simulink model "project_task3"  (R2020b)
settings: Solver=ode4  StartTime=0.0  StopTime=1200  FixedStep=0.001  RelTol=1e-3
model workspace (MAT data in the model file):
  A = Simulink.Parameter
  A.Value = Simulink.data.Expression
  A.Value.ExpressionString = "(Iw*4.68)/(5*Kt*r)"
  A.DataType = 'auto'
  A.Dimensions = -1
  B = Simulink.Parameter
  B.Value = Simulink.data.Expression
  B.Value.ExpressionString = "(mt*r*4.68)/(5*Kt)"
  B.DataType = 'auto'
  B.Dimensions = -1
  C_prime = Simulink.Parameter
  C_prime.Value = Simulink.data.Expression
  C_prime.Value.ExpressionString = "(mt*10*r*4.68)/(5*Kt)"
  C_prime.DataType = 'auto'
  C_prime.Dimensions = -1
  D = Simulink.Parameter
  D.Value = Simulink.data.Expression
  D.Value.ExpressionString = "5*Kv/r"
  D.DataType = 'auto'
  D.Dimensions = -1
  Iw = Simulink.Parameter
  Iw.Value = Simulink.data.Expression
  Iw.Value.ExpressionString = "mw*r^2"
  Iw.DataType = 'auto'
  Iw.Dimensions = -1
  Kt = 0.0758
  Kv = 0.076
  mb = 0.4
  mc = 0.2
  mm = 0.34
  mt = Simulink.Parameter
  mt.Value = Simulink.data.Expression
  mt.Value.ExpressionString = "mc+mb+mw+mm"
  mt.DataType = 'auto'
  mt.Dimensions = -1
  mw = Simulink.Parameter
  mw.Value = Simulink.data.Expression
  mw.Value.ExpressionString = "0.5*r"
  mw.DataType = 'auto'
  mw.Dimensions = -1
  r = 0.39
  y_dot_desired = 0.5
libraries: eePwmGenerator x1, simulink_extras x1
settings Model: OrderedModelArguments=off  Creator=melih.turkseven  LastModifiedBy=berkt
settings SFSimCC: CustomCodeUndefinedFunction=UseInterfaceOnly

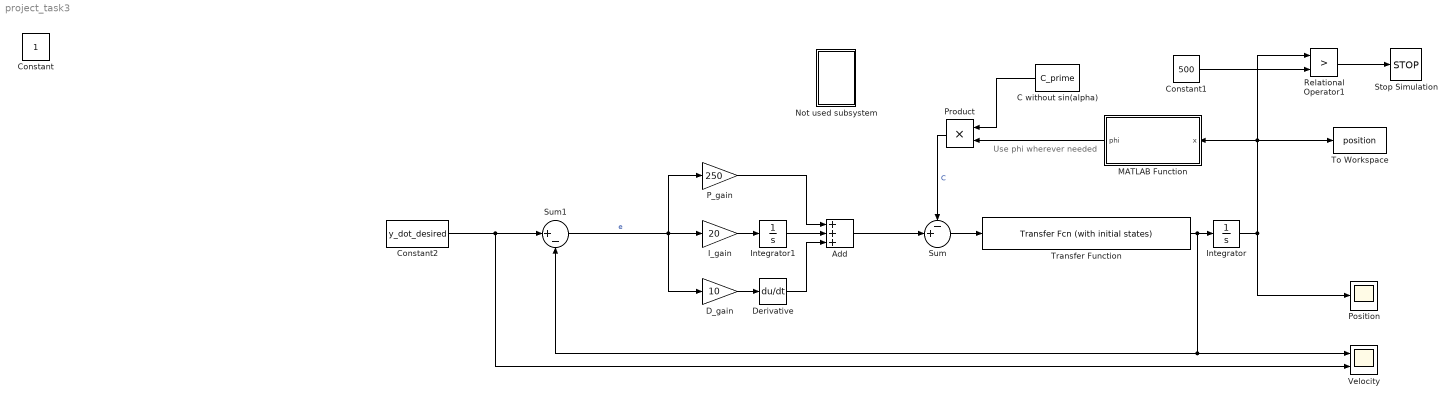
== system project_task3 ==
  note: Use phi wherever needed
  Add : Sum  Inputs=+++
  C without sin(alpha) : Constant  Value=C_prime
  Constant1 : Constant  Value=500
  Constant2 : Constant  Value=y_dot_desired
  D_gain : Gain  Gain=10
  Derivative : Derivative
  I_gain : Gain  Gain=20
  Integrator : Integrator
  Integrator1 : Integrator
  MATLAB Function : MATLAB Function  TreatAsAtomicUnit=on
  Not used subsystem : Subsystem
  P_gain : Gain  Gain=250
  Position : Scope
  Product : Product
  Relational Operator1 : RelationalOperator  Operator=>  OutDataTypeStr=boolean  RndMeth=Simplest
  Stop Simulation : Stop
  Sum : Sum  Inputs=-+|
  Sum1 : Sum  Inputs=|+-
  To Workspace : ToWorkspace  VariableName=position  SampleTime=-1
  Transfer Function : simulink_extras/Additional Linear/Transfer Fcn (with initial states)  N=[1]  D=[(A+B) D]  X0=0
  Velocity : Scope  NumInputPorts=2
  Constant : Constant  IOType=siggen
  wires:
  Transfer Function/1 -> Sum1/2, Velocity/1, Integrator/1
  MATLAB Function/1(phi) -> Product/2
  Relational Operator1/1 -> Stop Simulation/1
  Constant1/1 -> Relational Operator1/2
  Sum/1 -> Transfer Function/1
  C without sin(alpha)/1 -> Product/1
  Product/1 -> Sum/1  "C"
  Integrator/1 -> MATLAB Function/1(x), Relational Operator1/1, To Workspace/1, Position/1
  Constant2/1 -> Velocity/2, Sum1/1
  Sum1/1 -> P_gain/1, D_gain/1, I_gain/1  "e"
  I_gain/1 -> Integrator1/1
  D_gain/1 -> Derivative/1
  P_gain/1 -> Add/1
  Integrator1/1 -> Add/2
  Derivative/1 -> Add/3
  Add/1 -> Sum/2

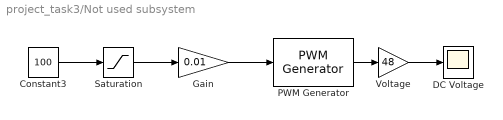
== system project_task3/Not used subsystem ==
  Constant3 : Constant  Value=100
  DC Voltage : Scope
  Gain : Gain  Gain=0.01
  PWM Generator : eePwmGenerator/PWM Generator  CarrCount=Up  Tper=0.01  Ts=0.001
  Saturation : Saturate  UpperLimit=100  LowerLimit=0
  Voltage : Gain  Gain=48
  wires:
  Saturation/1 -> Gain/1
  PWM Generator/1 -> Voltage/1
  Gain/1 -> PWM Generator/1
  Voltage/1 -> DC Voltage/1
  Constant3/1 -> Saturation/1

== matlab function project_task3/MATLAB Function ==
  data: x input; phi output
function phi = getInclination(x)

if x < 250
    phi = 0;
else
    if x < 350
        phi = sin(pi / 6);
    else
        phi = sin(pi / 18);
    end
end
